simulink model "FRControllerDubinsBoatOriginal"  (R2018a)
settings: Solver=VariableStepAuto  StartTime=0.0  StopTime=150  RelTol=1e-3
settings Model: Creator=KvonEllenrieder  LastModifiedBy=thedoctor
settings CodeAppCC: StateflowObjectComments=on

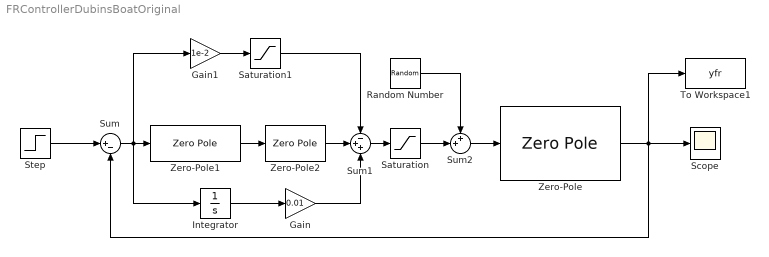
== system FRControllerDubinsBoatOriginal ==
  Gain : Gain  Gain=0.01
  Gain1 : Gain  Gain=1e-2
  Integrator : Integrator
  Random Number : RandomNumber  Mean=pi/36  Variance=pi/120  SampleTime=0.1
  Saturation : Saturate  UpperLimit=pi/6  LowerLimit=-pi/6
  Saturation1 : Saturate  UpperLimit=pi/6  LowerLimit=-pi/6
  Scope : Scope
  Step : Step  Time=10  After=4  SampleTime=0
  Sum : Sum  Inputs=|+-
  Sum1 : Sum  Inputs=-++
  Sum2 : Sum  Inputs=++|
  To Workspace1 : ToWorkspace  VariableName=yfr  SaveFormat=Timeseries  SampleTime=-1
  Zero-Pole : ZeroPole  Zeros=[]  Poles=[0 0 -5/4]  Gain=1.5
  Zero-Pole1 : ZeroPole  Zeros=-0.25  Poles=-16  Gain=55
  Zero-Pole2 : ZeroPole  Zeros=[]  Poles=[-3]
  wires:
  Zero-Pole/1 -> Sum/2, To Workspace1/1, Scope/1
  Step/1 -> Sum/1
  Sum/1 -> Gain1/1, Integrator/1, Zero-Pole1/1
  Saturation/1 -> Sum2/2
  Sum2/1 -> Zero-Pole/1
  Random Number/1 -> Sum2/1
  Zero-Pole1/1 -> Zero-Pole2/1
  Saturation1/1 -> Sum1/1
  Zero-Pole2/1 -> Sum1/2
  Sum1/1 -> Saturation/1
  Gain1/1 -> Saturation1/1
  Integrator/1 -> Gain/1
  Gain/1 -> Sum1/3
